simulink model "gm_detect_rising_edge"  (R2017a)
settings: Solver=FixedStepAuto  StartTime=0.0  StopTime=3  RelTol=1e-3
libraries: simulink x1
settings Model: Creator=mini  LastModifiedBy=mini
settings OptimizationCC: BlockReduction=off  ConditionallyExecuteInputs=off
settings DebuggingCC: InheritedTsInSrcMsg=none  SingleTaskRateTransMsg=error

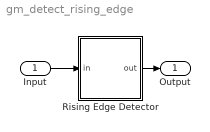
== system gm_detect_rising_edge ==
  Input : Inport  OutDataTypeStr=boolean
  Rising Edge Detector : Subsystem
  Output : Outport  OutDataTypeStr=boolean
  wires:
  Rising Edge Detector/1(out) -> Output/1
  Input/1 -> Rising Edge Detector/1(in)

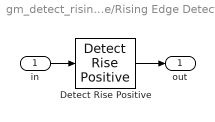
== system gm_detect_rising_edge/Rising Edge Detector ==
  in : Inport  OutDataTypeStr=boolean
  Detect Rise Positive : simulink/Logic and Bit Operations/Detect Rise Positive  vinit=0  OutDataTypeStr=boolean
  out : Outport  OutDataTypeStr=boolean
  wires:
  Detect Rise Positive/1 -> out/1
  in/1 -> Detect Rise Positive/1
